simulink model "Simulink_5"  (R2016b)
settings: Solver=VariableStepAuto  StartTime=0.0  StopTime=50  RelTol=1e-3
values from neighbouring files (symbols this model uses):
  C_lat = [1 0 0 0 ... (first row only)    [ejercicio07_lateral_C.m]
  D_lat = zeros(2)    [ejercicio07_lateral_C.m]
  dt = 0.001    [ejercicio07_lateral_C.m]    (also in ejercicio07_longitudinal_C.m)
  F_lat = A_lat*Tm + I    [ejercicio07_lateral_C.m]
  G_lat = B_lat*Tm    [ejercicio07_lateral_C.m]
  Kc = Kc_a(:,1:4)    [ejercicio07_lateral_C.m]    (also in ejercicio07_longitudinal_C.m)
  Ki = -Kc_a(:,5:6)    [ejercicio07_lateral_C.m]    (also in ejercicio07_longitudinal_C.m)
  Ko_d = dlqe(F_lat,G_lat,C_lat,V1,V2)    [ejercicio07_lateral_C.m]    (also in ejercicio07_longitudinal_C.m = dlqe(F_lon,G_lon,C_lon,V1,V2))
  PreC = [Cyr*(I-Fyr)^(-1)*G_lat+D_lat]^(-1)    [ejercicio07_lateral_C.m]    (also in ejercicio07_longitudinal_C.m = [Cyr*(I-Fyr)^(-1)*G_lon+D_lon]^(-1))
  tau_a = 0.5    [ejercicio07_lateral_C.m]
  tau_r = 1/20    (= 0.05)    [ejercicio07_lateral_C.m]
  Tm = 0.003    [ejercicio07_lateral_C.m]    (also in ejercicio07_longitudinal_C.m)
undefined symbols (not defined in the file or in its folder): DiscIntNeverNeededParam, Ko
undefined symbols (not defined in the file): sys_lat
(part 1 of 2)
settings Model: Creator=mluser  LastModifiedBy=Alvaro
settings DataIOCC: ReturnWorkspaceOutputs=on
settings DebuggingCC: SFMachineParentedDataDiag=error
settings SFSimCC: SimUseLocalCustomCode=on
settings RTWCC: RTWUseLocalCustomCode=on

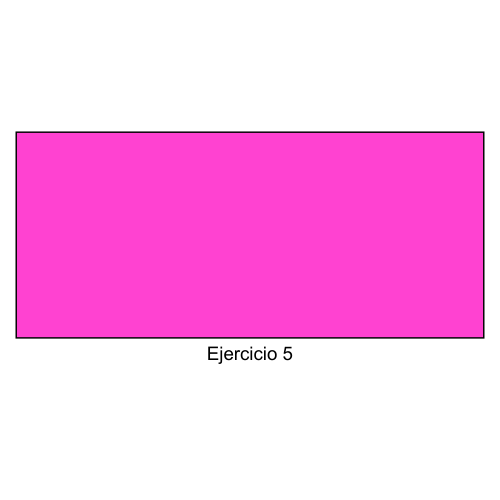
[thumbnail: Simulink's stored preview of the top-level diagram]
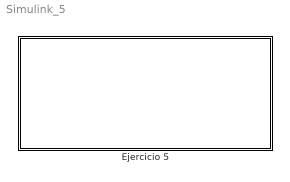
== system Simulink_5 ==
  Ejercicio 5 : Subsystem

== system Simulink_5/Ejercicio 5 ==
  EJERCICIO 5 CONTINUO : Subsystem  Commented=on
  EJERCICIO 5 DISCRETO : Subsystem  Commented=on

== system Simulink_5/Ejercicio 5/EJERCICIO 5 CONTINUO ==
  Control lateral con observador de estados %bien : Subsystem
  Control lateral con observador de estados sin perturbacion %bien : Subsystem
  Control laterall con accion integral %bien : Subsystem

== system Simulink_5/Ejercicio 5/EJERCICIO 5 DISCRETO ==
  COMPARATIVA : Subsystem
  CONTROL LATERAL DISCRETO : Subsystem  Commented=on
  CONTROL LATERAL DISCRETO ACCION INTEGRAL : Subsystem  Commented=on
  CONTROL LATERALDISCRETO FBW : Subsystem  Commented=on

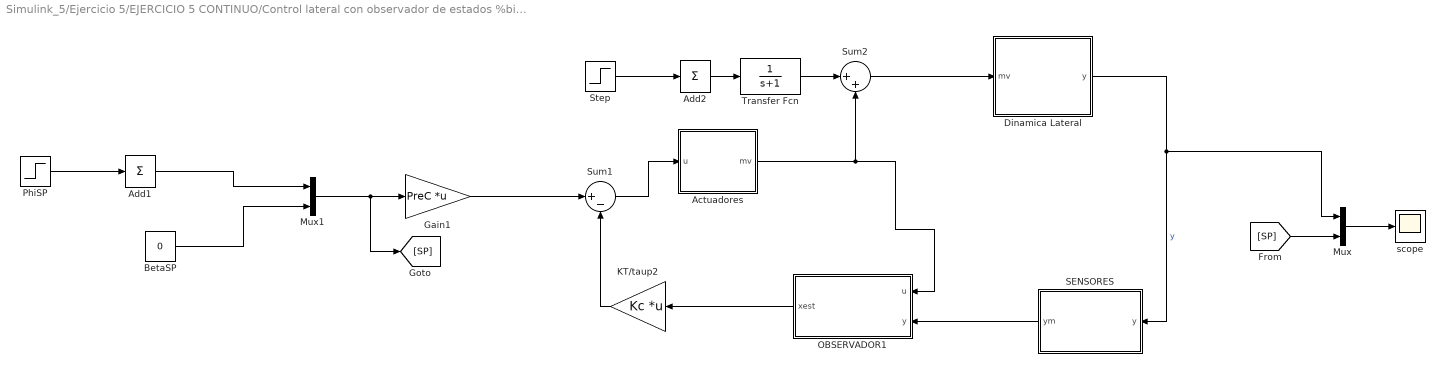
== system Simulink_5/Ejercicio 5/EJERCICIO 5 CONTINUO/Control lateral con observador de estados %bien ==
  Actuadores : Subsystem
  Add1 : Sum  Inputs=+
  Add2 : Sum  Inputs=+
  BetaSP : Constant  Value=0
  Dinamica Lateral : Subsystem  mask(Dinámica longitudinal F-16){A=sys_lat.a, B=sys_lat.b, C=sys_lat.c, D=sys_lat.d, X0=[0 0 0 0]}
      mask prompts: A "Matriz de estados (A)"; B "Matriz de entrada (B)"; C "Matriz de salida (C)"; D "Matriz de transmisión directa (D)"; X0 "Condiciones iniciales (nominales)"
      mask help: Modelo lineal de la dinámica longitudinal del F-16
  Gain1 : Gain  Gain=PreC  Multiplication=Matrix(K*u)
  KT/taup2 : Gain  Gain=Kc  Multiplication=Matrix(K*u)
  Mux : Mux  Inputs=2
  Mux1 : Mux  Inputs=2
  OBSERVADOR1 : Subsystem  mask(Dinámica longitudinal F-16){A=sys_lat.a, B=sys_lat.b, C=sys_lat.c, D=sys_lat.d, X0=[0 0 0 0], Ko=Ko}
      mask prompts: A "Matriz de estados (A)"; B "Matriz de entrada (B)"; C "Matriz de salida (C)"; D "Matriz de transmisión directa (D)"; X0 "Condiciones iniciales (nominales)"; Ko "Ganancia del observador"
      mask help: Modelo lineal de la dinámica longitudinal del F-16
  PhiSP : Step  Time=[5 25]  Before=[0 0]  After=[10 -10]  SampleTime=0
  SENSORES : Subsystem
  Step : Step  Time=[40 41]  After=[1 -1]  SampleTime=0
  Sum1 : Sum  Inputs=|+-
  Sum2 : Sum  Inputs=|++
  Transfer Fcn : TransferFcn  Denominator=[1 1]
  scope : Scope
  wires:
  Mux1/1 -> [SP], Gain1/1
  Gain1/1 -> Sum1/1
  Mux/1 -> scope/1
  [SP] -> Mux/2
  KT/taup2/1 -> Sum1/2
  SENSORES/1(ym) -> OBSERVADOR1/2(y)
  OBSERVADOR1/1(xest) -> KT/taup2/1
  Dinamica Lateral/1(y) -> Mux/1, SENSORES/1(y)  "y"
  PhiSP/1 -> Add1/1
  Add1/1 -> Mux1/1
  Actuadores/1(mv) -> OBSERVADOR1/1(u), Sum2/2
  Sum1/1 -> Actuadores/1(u)
  BetaSP/1 -> Mux1/2
  Step/1 -> Add2/1
  Transfer Fcn/1 -> Sum2/1
  Add2/1 -> Transfer Fcn/1
  Sum2/1 -> Dinamica Lateral/1(mv)

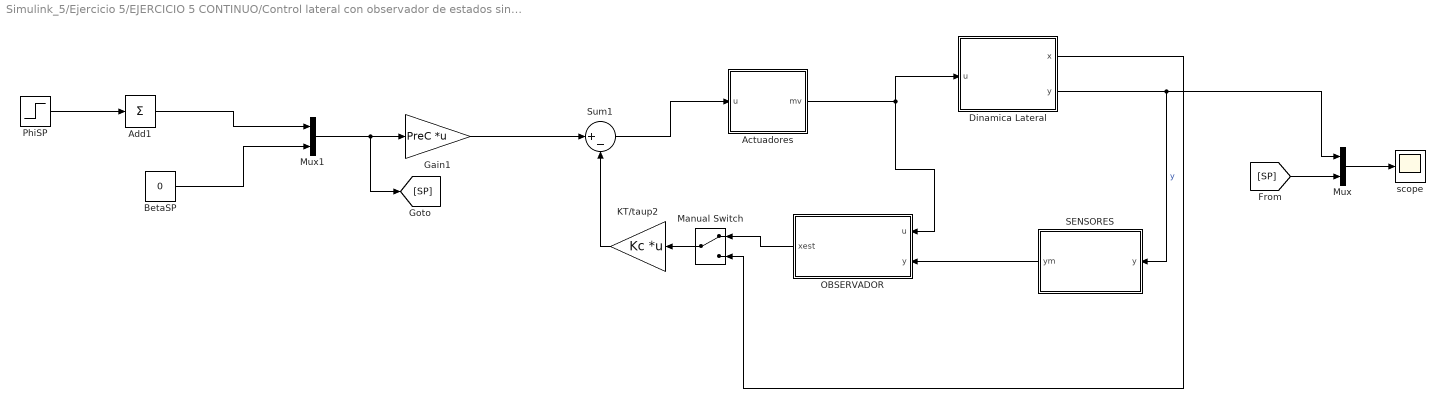
== system Simulink_5/Ejercicio 5/EJERCICIO 5 CONTINUO/Control lateral con observador de estados sin perturbacion %bien ==
  Actuadores : Subsystem
  Add1 : Sum  Inputs=+
  BetaSP : Constant  Value=0
  Dinamica Lateral : Subsystem  mask(Dinámica longitudinal F-16){A=sys_lat.a, B=sys_lat.b, C=sys_lat.c, D=sys_lat.d, X0=[0 0 0 0]}
      mask prompts: A "Matriz de estados (A)"; B "Matriz de entrada (B)"; C "Matriz de salida (C)"; D "Matriz de transmisión directa (D)"; X0 "Condiciones iniciales (nominales)"
      mask help: Modelo lineal de la dinámica longitudinal del F-16
  Gain1 : Gain  Gain=PreC  Multiplication=Matrix(K*u)
  KT/taup2 : Gain  Gain=Kc  Multiplication=Matrix(K*u)
  Manual Switch : ManualSwitch
  Mux : Mux  Inputs=2
  Mux1 : Mux  Inputs=2
  OBSERVADOR : Subsystem  mask(Dinámica longitudinal F-16){A=sys_lat.a, B=sys_lat.b, C=sys_lat.c, D=sys_lat.d, X0=[0 0 0 0], Ko=Ko}
      mask prompts: A "Matriz de estados (A)"; B "Matriz de entrada (B)"; C "Matriz de salida (C)"; D "Matriz de transmisión directa (D)"; X0 "Condiciones iniciales (nominales)"; Ko "Ganancia del observador"
      mask help: Modelo lineal de la dinámica longitudinal del F-16
  PhiSP : Step  Time=[5 25]  Before=[0 0]  After=[10 -10]  SampleTime=0
  SENSORES : Subsystem
  Sum1 : Sum  Inputs=|+-
  scope : Scope
  wires:
  Actuadores/1(mv) -> Dinamica Lateral/1(u), OBSERVADOR/1(u)
  [SP] -> Mux/2
  Dinamica Lateral/2(y) -> Mux/1, SENSORES/1(y)  "y"
  Add1/1 -> Mux1/1
  Mux/1 -> scope/1
  BetaSP/1 -> Mux1/2
  PhiSP/1 -> Add1/1
  Gain1/1 -> Sum1/1
  KT/taup2/1 -> Sum1/2
  Sum1/1 -> Actuadores/1(u)
  SENSORES/1(ym) -> OBSERVADOR/2(y)
  Mux1/1 -> [SP], Gain1/1
  Manual Switch/1 -> KT/taup2/1
  OBSERVADOR/1(xest) -> Manual Switch/1
  Dinamica Lateral/1(x) -> Manual Switch/2

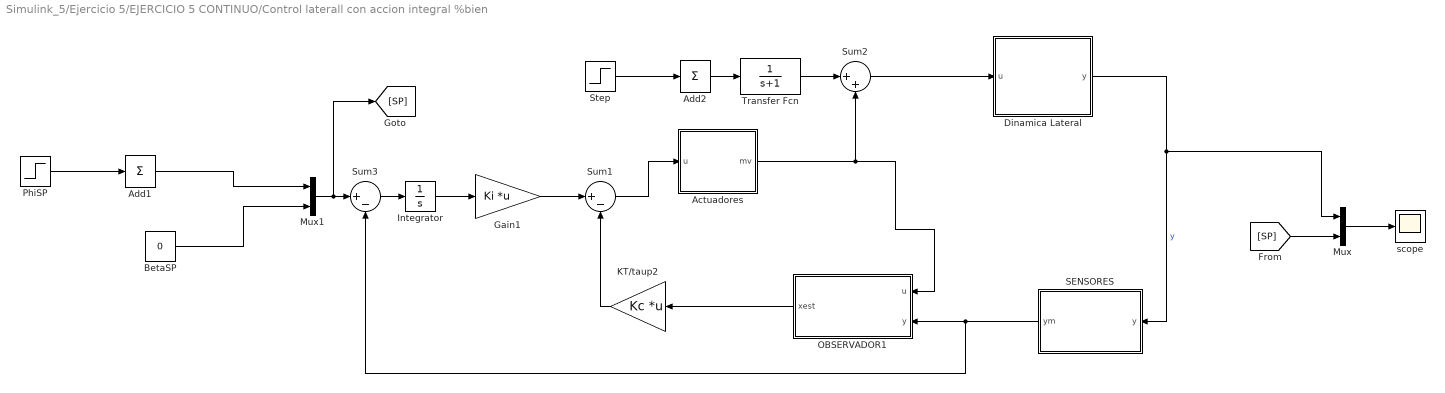
== system Simulink_5/Ejercicio 5/EJERCICIO 5 CONTINUO/Control laterall con accion integral %bien ==
  Actuadores : Subsystem
  Add1 : Sum  Inputs=+
  Add2 : Sum  Inputs=+
  BetaSP : Constant  Value=0
  Dinamica Lateral : Subsystem  mask(Dinámica longitudinal F-16){A=sys_lat.a, B=sys_lat.b, C=sys_lat.c, D=sys_lat.d, X0=[0 0 0 0]}
      mask prompts: A "Matriz de estados (A)"; B "Matriz de entrada (B)"; C "Matriz de salida (C)"; D "Matriz de transmisión directa (D)"; X0 "Condiciones iniciales (nominales)"
      mask help: Modelo lineal de la dinámica longitudinal del F-16
  Gain1 : Gain  Gain=Ki  Multiplication=Matrix(K*u)
  Integrator : Integrator
  KT/taup2 : Gain  Gain=Kc  Multiplication=Matrix(K*u)
  Mux : Mux  Inputs=2
  Mux1 : Mux  Inputs=2
  OBSERVADOR1 : Subsystem  mask(Dinámica longitudinal F-16){A=sys_lat.a, B=sys_lat.b, C=sys_lat.c, D=sys_lat.d, X0=[0 0 0 0], Ko=Ko}
      mask prompts: A "Matriz de estados (A)"; B "Matriz de entrada (B)"; C "Matriz de salida (C)"; D "Matriz de transmisión directa (D)"; X0 "Condiciones iniciales (nominales)"; Ko "Ganancia del observador"
      mask help: Modelo lineal de la dinámica longitudinal del F-16
  PhiSP : Step  Time=[5 25]  Before=[0 0]  After=[10 -10]  SampleTime=0
  SENSORES : Subsystem
  Step : Step  Time=[40 41]  After=[1 -1]  SampleTime=0
  Sum1 : Sum  Inputs=|+-
  Sum2 : Sum  Inputs=|++
  Sum3 : Sum  Inputs=|+-
  Transfer Fcn : TransferFcn  Denominator=[1 1]
  scope : Scope
  wires:
  Actuadores/1(mv) -> OBSERVADOR1/1(u), Sum2/2
  Dinamica Lateral/1(y) -> Mux/1, SENSORES/1(y)  "y"
  BetaSP/1 -> Mux1/2
  Add1/1 -> Mux1/1
  Sum2/1 -> Dinamica Lateral/1(u)
  KT/taup2/1 -> Sum1/2
  Gain1/1 -> Sum1/1
  Add2/1 -> Transfer Fcn/1
  Step/1 -> Add2/1
  PhiSP/1 -> Add1/1
  SENSORES/1(ym) -> OBSERVADOR1/2(y), Sum3/2
  Mux/1 -> scope/1
  Sum1/1 -> Actuadores/1(u)
  [SP] -> Mux/2
  OBSERVADOR1/1(xest) -> KT/taup2/1
  Transfer Fcn/1 -> Sum2/1
  Mux1/1 -> [SP], Sum3/1
  Integrator/1 -> Gain1/1
  Sum3/1 -> Integrator/1

== system Simulink_5/Ejercicio 5/EJERCICIO 5 DISCRETO/COMPARATIVA ==
  Comparativa Integral : Subsystem  Commented=on
  Comparativa modal : Subsystem

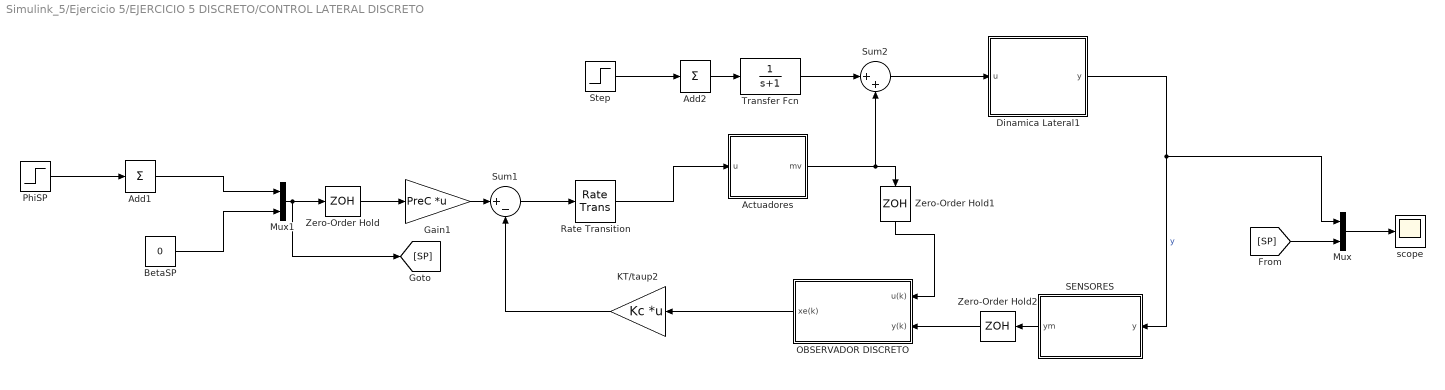
== system Simulink_5/Ejercicio 5/EJERCICIO 5 DISCRETO/CONTROL LATERAL DISCRETO ==
  Actuadores : Subsystem
  Add1 : Sum  Inputs=+
  Add2 : Sum  Inputs=+
  BetaSP : Constant  Value=0
  Dinamica Lateral1 : Subsystem  mask(Dinámica longitudinal F-16){A=sys_lat.a, B=sys_lat.b, C=sys_lat.c, D=sys_lat.d, X0=[0 0 0 0]}
      mask prompts: A "Matriz de estados (A)"; B "Matriz de entrada (B)"; C "Matriz de salida (C)"; D "Matriz de transmisión directa (D)"; X0 "Condiciones iniciales (nominales)"
      mask help: Modelo lineal de la dinámica longitudinal del F-16
  Gain1 : Gain  Gain=PreC  Multiplication=Matrix(K*u)
  KT/taup2 : Gain  Gain=Kc  Multiplication=Matrix(K*u)
  Mux : Mux  Inputs=2
  Mux1 : Mux  Inputs=2
  OBSERVADOR DISCRETO : Subsystem  mask(Dinámica longitudinal F-16){F=F_lat, G=G_lat, C=C_lat, D=D_lat, Ko=Ko_d}
      mask prompts: F "Matriz de estados (A)"; G "Matriz de entrada (B)"; C "Matriz de salida (C)"; D "Matriz de transmisión directa (D)"; Ko "Ganancia del observador"
      mask help: Modelo lineal de la dinámica longitudinal del F-16
  PhiSP : Step  Time=[5 25]  Before=[0 0]  After=[10 -10]  SampleTime=0
  Rate Transition : RateTransition
  SENSORES : Subsystem
  Step : Step  Time=[40 41]  After=[1 -1]  SampleTime=0
  Sum1 : Sum  Inputs=|+-
  Sum2 : Sum  Inputs=|++
  Transfer Fcn : TransferFcn  Denominator=[1 1]
  Zero-Order Hold : ZeroOrderHold  SampleTime=-1
  Zero-Order Hold1 : ZeroOrderHold  SampleTime=-1
  Zero-Order Hold2 : ZeroOrderHold  SampleTime=-1
  scope : Scope
  wires:
  Actuadores/1(mv) -> Zero-Order Hold1/1, Sum2/2
  Mux1/1 -> Zero-Order Hold/1, [SP]
  [SP] -> Mux/2
  Add1/1 -> Mux1/1
  OBSERVADOR DISCRETO/1(xe(k)) -> KT/taup2/1
  SENSORES/1(ym) -> Zero-Order Hold2/1
  KT/taup2/1 -> Sum1/2
  PhiSP/1 -> Add1/1
  Gain1/1 -> Sum1/1
  Mux/1 -> scope/1
  BetaSP/1 -> Mux1/2
  Dinamica Lateral1/1(y) -> SENSORES/1(y), Mux/1  "y"
  Zero-Order Hold/1 -> Gain1/1
  Rate Transition/1 -> Actuadores/1(u)
  Sum1/1 -> Rate Transition/1
  Zero-Order Hold1/1 -> OBSERVADOR DISCRETO/1(u(k))
  Zero-Order Hold2/1 -> OBSERVADOR DISCRETO/2(y(k))
  Add2/1 -> Transfer Fcn/1
  Step/1 -> Add2/1
  Transfer Fcn/1 -> Sum2/1
  Sum2/1 -> Dinamica Lateral1/1(u)

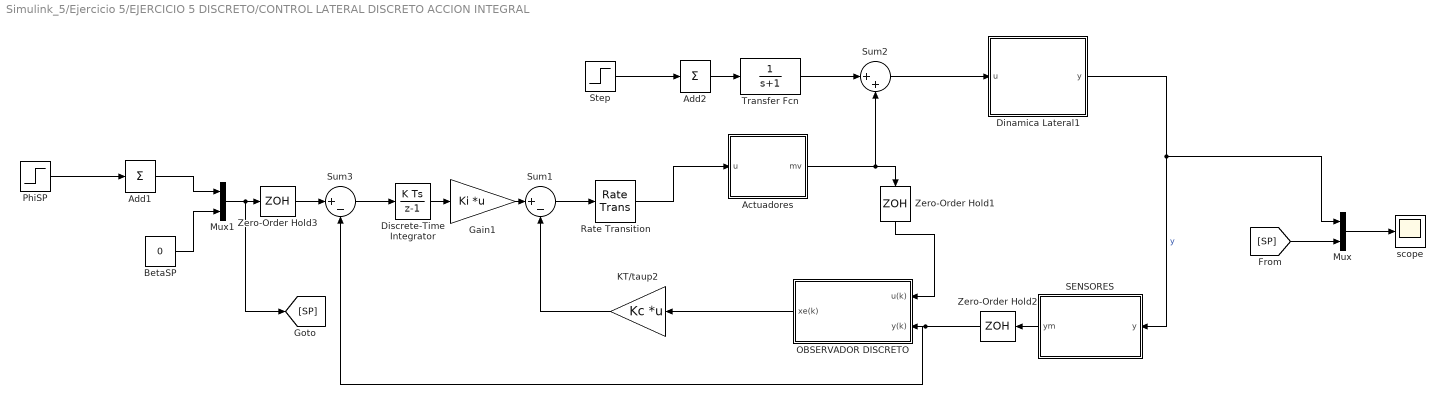
== system Simulink_5/Ejercicio 5/EJERCICIO 5 DISCRETO/CONTROL LATERAL DISCRETO ACCION INTEGRAL ==
  Actuadores : Subsystem
  Add1 : Sum  Inputs=+
  Add2 : Sum  Inputs=+
  BetaSP : Constant  Value=0
  Dinamica Lateral1 : Subsystem  mask(Dinámica longitudinal F-16){A=sys_lat.a, B=sys_lat.b, C=sys_lat.c, D=sys_lat.d, X0=[0 0 0 0]}
      mask prompts: A "Matriz de estados (A)"; B "Matriz de entrada (B)"; C "Matriz de salida (C)"; D "Matriz de transmisión directa (D)"; X0 "Condiciones iniciales (nominales)"
      mask help: Modelo lineal de la dinámica longitudinal del F-16
  Discrete-Time Integrator : DiscreteIntegrator  InitialConditionSetting=State (most efficient)  SampleTime=-1  ICPrevOutput=DiscIntNeverNeededParam  ICPrevScaledInput=DiscIntNeverNeededParam
  Gain1 : Gain  Gain=Ki  Multiplication=Matrix(K*u)
  KT/taup2 : Gain  Gain=Kc  Multiplication=Matrix(K*u)
  Mux : Mux  Inputs=2
  Mux1 : Mux  Inputs=2
  OBSERVADOR DISCRETO : Subsystem  mask(Dinámica longitudinal F-16){F=F_lat, G=G_lat, C=C_lat, D=D_lat, Ko=Ko_d}
      mask prompts: F "Matriz de estados (A)"; G "Matriz de entrada (B)"; C "Matriz de salida (C)"; D "Matriz de transmisión directa (D)"; Ko "Ganancia del observador"
      mask help: Modelo lineal de la dinámica longitudinal del F-16
  PhiSP : Step  Time=[5 25]  Before=[0 0]  After=[10 -10]  SampleTime=0
  Rate Transition : RateTransition
  SENSORES : Subsystem
  Step : Step  Time=[40 41]  After=[1 -1]  SampleTime=0
  Sum1 : Sum  Inputs=|+-
  Sum2 : Sum  Inputs=|++
  Sum3 : Sum  Inputs=|+-
  Transfer Fcn : TransferFcn  Denominator=[1 1]
  Zero-Order Hold1 : ZeroOrderHold  SampleTime=-1
  Zero-Order Hold2 : ZeroOrderHold  SampleTime=-1
  Zero-Order Hold3 : ZeroOrderHold  SampleTime=-1
  scope : Scope
  wires:
  Zero-Order Hold2/1 -> Sum3/2, OBSERVADOR DISCRETO/2(y(k))
  Rate Transition/1 -> Actuadores/1(u)
  Mux1/1 -> Zero-Order Hold3/1, [SP]
  Dinamica Lateral1/1(y) -> SENSORES/1(y), Mux/1  "y"
  [SP] -> Mux/2
  Add2/1 -> Transfer Fcn/1
  Gain1/1 -> Sum1/1
  Discrete-Time Integrator/1 -> Gain1/1
  SENSORES/1(ym) -> Zero-Order Hold2/1
  Transfer Fcn/1 -> Sum2/1
  Step/1 -> Add2/1
  KT/taup2/1 -> Sum1/2
  BetaSP/1 -> Mux1/2
  Sum1/1 -> Rate Transition/1
  OBSERVADOR DISCRETO/1(xe(k)) -> KT/taup2/1
  Add1/1 -> Mux1/1
  Actuadores/1(mv) -> Zero-Order Hold1/1, Sum2/2
  PhiSP/1 -> Add1/1
  Mux/1 -> scope/1
  Sum2/1 -> Dinamica Lateral1/1(u)
  Zero-Order Hold1/1 -> OBSERVADOR DISCRETO/1(u(k))
  Sum3/1 -> Discrete-Time Integrator/1
  Zero-Order Hold3/1 -> Sum3/1

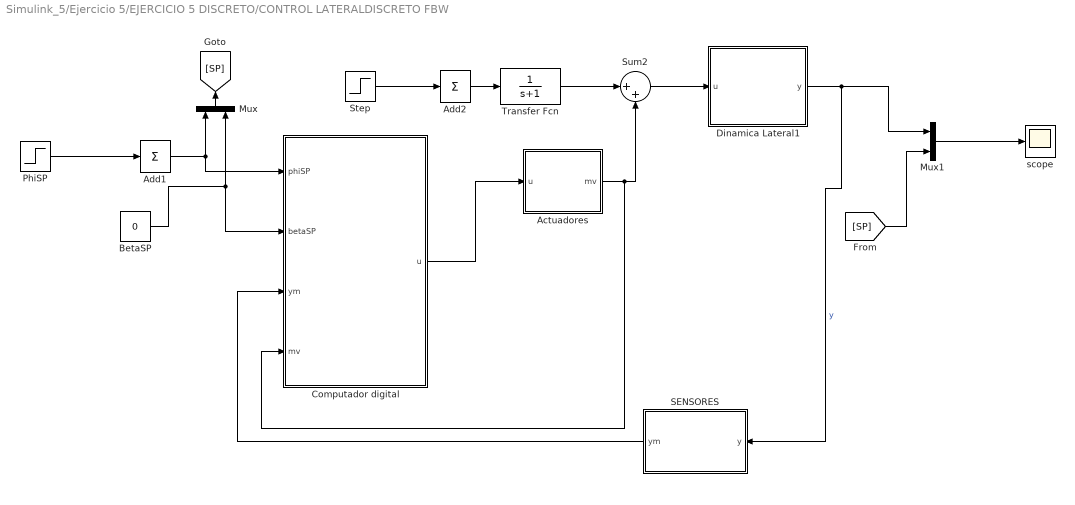
== system Simulink_5/Ejercicio 5/EJERCICIO 5 DISCRETO/CONTROL LATERALDISCRETO FBW ==
  Actuadores : Subsystem
  Add1 : Sum  Inputs=+
  Add2 : Sum  Inputs=+
  BetaSP : Constant  Value=0
  Computador digital : Subsystem
  Dinamica Lateral1 : Subsystem  mask(Dinámica longitudinal F-16){A=sys_lat.a, B=sys_lat.b, C=sys_lat.c, D=sys_lat.d, X0=[0 0 0 0]}
      mask prompts: A "Matriz de estados (A)"; B "Matriz de entrada (B)"; C "Matriz de salida (C)"; D "Matriz de transmisión directa (D)"; X0 "Condiciones iniciales (nominales)"
      mask help: Modelo lineal de la dinámica longitudinal del F-16
  Mux : Mux  Inputs=2
  Mux1 : Mux  Inputs=2
  PhiSP : Step  Time=[5 25]  Before=[0 0]  After=[10 -10]  SampleTime=0
  SENSORES : Subsystem
  Step : Step  Time=[40 41]  After=[1 -1]  SampleTime=0
  Sum2 : Sum  Inputs=|++
  Transfer Fcn : TransferFcn  Denominator=[1 1]
  scope : Scope
  wires:
  Add1/1 -> Computador digital/1(phiSP), Mux/1
  BetaSP/1 -> Computador digital/2(betaSP), Mux/2
  PhiSP/1 -> Add1/1
  Transfer Fcn/1 -> Sum2/1
  Add2/1 -> Transfer Fcn/1
  Sum2/1 -> Dinamica Lateral1/1(u)
  Step/1 -> Add2/1
  Actuadores/1(mv) -> Computador digital/4(mv), Sum2/2
  Mux/1 -> [SP]
  Mux1/1 -> scope/1
  [SP] -> Mux1/2
  Dinamica Lateral1/1(y) -> SENSORES/1(y), Mux1/1  "y"
  Computador digital/1(u) -> Actuadores/1(u)
  SENSORES/1(ym) -> Computador digital/3(ym)

== system Simulink_5/Ejercicio 5/EJERCICIO 5 CONTINUO/Control lateral con observador de estados %bien/Actuadores ==
  u : Inport
  Aleron : Subsystem
  Demux : Demux  Outputs=2
  Mux2 : Mux  Inputs=2
  Scope : Scope
  TIMÓN : Subsystem
  mv : Outport
  wires:
  u/1 -> Demux/1
  Mux2/1 -> mv/1, Scope/1
  Demux/1 -> Aleron/1(u_a)
  Demux/2 -> TIMÓN/1(u_r)
  Aleron/1(delta_a) -> Mux2/1
  TIMÓN/1(delta_r) -> Mux2/2

== system Simulink_5/Ejercicio 5/EJERCICIO 5 CONTINUO/Control lateral con observador de estados %bien/Dinamica Lateral ==
  mv : Inport
  Integrator5 : Integrator
  Km1 : Gain  Gain=D  Multiplication=Matrix(K*u)
  Km10 : Gain  Gain=A  Multiplication=Matrix(K*u)
  Km2 : Gain  Gain=C  Multiplication=Matrix(K*u)
  Km8 : Gain  Gain=B  Multiplication=Matrix(K*u)
  Sum1 : Sum  Inputs=++|
  Sum12 : Sum  Inputs=|++
  y : Outport
  wires:
  Km8/1 -> Sum12/1
  Sum12/1 -> Integrator5/1
  Integrator5/1 -> Km10/1, Km2/1  "x"
  Km10/1 -> Sum12/2
  Km2/1 -> Sum1/2
  Km1/1 -> Sum1/1
  Sum1/1 -> y/1
  mv/1 -> Km8/1, Km1/1

== system Simulink_5/Ejercicio 5/EJERCICIO 5 CONTINUO/Control lateral con observador de estados %bien/OBSERVADOR1 ==
  u : Inport
  y : Inport  Port=2
  Integrator5 : Integrator
  Km1 : Gain  Gain=D  Multiplication=Matrix(K*u)
  Km10 : Gain  Gain=A  Multiplication=Matrix(K*u)
  Km2 : Gain  Gain=C  Multiplication=Matrix(K*u)
  Km3 : Gain  Gain=Ko  Multiplication=Matrix(K*u)
  Km8 : Gain  Gain=B  Multiplication=Matrix(K*u)
  Sum1 : Sum  Inputs=++|
  Sum12 : Sum  Inputs=+++
  Sum2 : Sum  Inputs=+-|
  xest : Outport
  wires:
  Km8/1 -> Sum12/1
  Sum12/1 -> Integrator5/1
  Integrator5/1 -> Km2/1, Km10/1, xest/1  "xe"
  Km10/1 -> Sum12/3
  Km2/1 -> Sum1/2
  Km1/1 -> Sum1/1
  Sum1/1 -> Sum2/2  "ye"
  u/1 -> Km8/1, Km1/1
  y/1 -> Sum2/1
  Sum2/1 -> Km3/1
  Km3/1 -> Sum12/2

== system Simulink_5/Ejercicio 5/EJERCICIO 5 CONTINUO/Control lateral con observador de estados %bien/SENSORES ==
  y : Inport
  Add2 : Sum
  Add3 : Sum
  Demux : Demux  Outputs=2
  Mux2 : Mux  Inputs=2
  Ruido de medida1 : RandomNumber  Variance=1e-6  Seed=123456  SampleTime=dt
  Ruido de medida2 : RandomNumber  Variance=1e-6  Seed=123456  SampleTime=dt
  ym : Outport
  wires:
  y/1 -> Demux/1
  Ruido de medida1/1 -> Add2/1
  Add2/1 -> Mux2/1
  Demux/1 -> Add2/2
  Mux2/1 -> ym/1
  Demux/2 -> Add3/1
  Add3/1 -> Mux2/2
  Ruido de medida2/1 -> Add3/2

== system Simulink_5/Ejercicio 5/EJERCICIO 5 CONTINUO/Control lateral con observador de estados sin perturbacion %bien/Actuadores ==
  u : Inport
  Aleron : Subsystem
  Demux : Demux  Outputs=2
  Mux2 : Mux  Inputs=2
  Scope : Scope
  TIMÓN : Subsystem
  mv : Outport
  wires:
  u/1 -> Demux/1
  Mux2/1 -> mv/1, Scope/1
  Demux/1 -> Aleron/1(u_a)
  Demux/2 -> TIMÓN/1(u_r)
  Aleron/1(delta_a) -> Mux2/1
  TIMÓN/1(delta_r) -> Mux2/2

== system Simulink_5/Ejercicio 5/EJERCICIO 5 CONTINUO/Control lateral con observador de estados sin perturbacion %bien/Dinamica Lateral ==
  u : Inport
  Integrator5 : Integrator
  Km1 : Gain  Gain=D  Multiplication=Matrix(K*u)
  Km10 : Gain  Gain=A  Multiplication=Matrix(K*u)
  Km2 : Gain  Gain=C  Multiplication=Matrix(K*u)
  Km8 : Gain  Gain=B  Multiplication=Matrix(K*u)
  Sum1 : Sum  Inputs=++|
  Sum12 : Sum  Inputs=|++
  x : Outport
  y : Outport  Port=2
  wires:
  Km8/1 -> Sum12/1
  Sum12/1 -> Integrator5/1
  Integrator5/1 -> x/1, Km10/1, Km2/1  "x"
  Km10/1 -> Sum12/2
  Km2/1 -> Sum1/2
  Km1/1 -> Sum1/1
  Sum1/1 -> y/1
  u/1 -> Km8/1, Km1/1

== system Simulink_5/Ejercicio 5/EJERCICIO 5 CONTINUO/Control lateral con observador de estados sin perturbacion %bien/OBSERVADOR ==
  u : Inport
  y : Inport  Port=2
  Integrator5 : Integrator
  Km1 : Gain  Gain=D  Multiplication=Matrix(K*u)
  Km10 : Gain  Gain=A  Multiplication=Matrix(K*u)
  Km2 : Gain  Gain=C  Multiplication=Matrix(K*u)
  Km3 : Gain  Gain=Ko  Multiplication=Matrix(K*u)
  Km8 : Gain  Gain=B  Multiplication=Matrix(K*u)
  Sum1 : Sum  Inputs=++|
  Sum12 : Sum  Inputs=+++
  Sum2 : Sum  Inputs=+-|
  xest : Outport
  wires:
  Km8/1 -> Sum12/1
  Sum12/1 -> Integrator5/1
  Integrator5/1 -> Km2/1, Km10/1, xest/1  "xe"
  Km10/1 -> Sum12/3
  Km2/1 -> Sum1/2
  Km1/1 -> Sum1/1
  Sum1/1 -> Sum2/2  "ye"
  u/1 -> Km8/1, Km1/1
  y/1 -> Sum2/1
  Sum2/1 -> Km3/1
  Km3/1 -> Sum12/2

== system Simulink_5/Ejercicio 5/EJERCICIO 5 CONTINUO/Control lateral con observador de estados sin perturbacion %bien/SENSORES ==
  y : Inport
  Add2 : Sum
  Add3 : Sum
  Demux : Demux  Outputs=2
  Mux2 : Mux  Inputs=2
  Ruido de medida1 : RandomNumber  Variance=1e-6  Seed=123456  SampleTime=dt
  Ruido de medida2 : RandomNumber  Variance=1e-6  Seed=123456  SampleTime=dt
  ym : Outport
  wires:
  y/1 -> Demux/1
  Ruido de medida1/1 -> Add2/1
  Add2/1 -> Mux2/1
  Demux/1 -> Add2/2
  Mux2/1 -> ym/1
  Demux/2 -> Add3/1
  Add3/1 -> Mux2/2
  Ruido de medida2/1 -> Add3/2

== system Simulink_5/Ejercicio 5/EJERCICIO 5 CONTINUO/Control laterall con accion integral %bien/Actuadores ==
  u : Inport
  Aleron : Subsystem
  Demux : Demux  Outputs=2
  Mux2 : Mux  Inputs=2
  Scope : Scope
  TIMÓN : Subsystem
  mv : Outport
  wires:
  u/1 -> Demux/1
  Mux2/1 -> mv/1, Scope/1
  Demux/1 -> Aleron/1(u_a)
  Demux/2 -> TIMÓN/1(u_r)
  Aleron/1(delta_a) -> Mux2/1
  TIMÓN/1(delta_r) -> Mux2/2

== system Simulink_5/Ejercicio 5/EJERCICIO 5 CONTINUO/Control laterall con accion integral %bien/Dinamica Lateral ==
  u : Inport
  Integrator5 : Integrator
  Km1 : Gain  Gain=D  Multiplication=Matrix(K*u)
  Km10 : Gain  Gain=A  Multiplication=Matrix(K*u)
  Km2 : Gain  Gain=C  Multiplication=Matrix(K*u)
  Km8 : Gain  Gain=B  Multiplication=Matrix(K*u)
  Sum1 : Sum  Inputs=++|
  Sum12 : Sum  Inputs=|++
  y : Outport
  wires:
  Km8/1 -> Sum12/1
  Sum12/1 -> Integrator5/1
  Integrator5/1 -> Km10/1, Km2/1  "x"
  Km10/1 -> Sum12/2
  Km2/1 -> Sum1/2
  Km1/1 -> Sum1/1
  Sum1/1 -> y/1
  u/1 -> Km8/1, Km1/1

== system Simulink_5/Ejercicio 5/EJERCICIO 5 CONTINUO/Control laterall con accion integral %bien/OBSERVADOR1 ==
  u : Inport
  y : Inport  Port=2
  Integrator5 : Integrator
  Km1 : Gain  Gain=D  Multiplication=Matrix(K*u)
  Km10 : Gain  Gain=A  Multiplication=Matrix(K*u)
  Km2 : Gain  Gain=C  Multiplication=Matrix(K*u)
  Km3 : Gain  Gain=Ko  Multiplication=Matrix(K*u)
  Km8 : Gain  Gain=B  Multiplication=Matrix(K*u)
  Sum1 : Sum  Inputs=++|
  Sum12 : Sum  Inputs=+++
  Sum2 : Sum  Inputs=+-|
  xest : Outport
  wires:
  Km8/1 -> Sum12/1
  Sum12/1 -> Integrator5/1
  Integrator5/1 -> Km2/1, Km10/1, xest/1  "xe"
  Km10/1 -> Sum12/3
  Km2/1 -> Sum1/2
  Km1/1 -> Sum1/1
  Sum1/1 -> Sum2/2  "ye"
  u/1 -> Km8/1, Km1/1
  y/1 -> Sum2/1
  Sum2/1 -> Km3/1
  Km3/1 -> Sum12/2

== system Simulink_5/Ejercicio 5/EJERCICIO 5 CONTINUO/Control laterall con accion integral %bien/SENSORES ==
  y : Inport
  Add2 : Sum
  Add3 : Sum
  Demux : Demux  Outputs=2
  Mux2 : Mux  Inputs=2
  Ruido de medida1 : RandomNumber  Variance=1e-6  Seed=123456  SampleTime=dt
  Ruido de medida2 : RandomNumber  Variance=1e-6  Seed=123456  SampleTime=dt
  ym : Outport
  wires:
  y/1 -> Demux/1
  Ruido de medida1/1 -> Add2/1
  Add2/1 -> Mux2/1
  Demux/1 -> Add2/2
  Mux2/1 -> ym/1
  Demux/2 -> Add3/1
  Add3/1 -> Mux2/2
  Ruido de medida2/1 -> Add3/2

== system Simulink_5/Ejercicio 5/EJERCICIO 5 DISCRETO/COMPARATIVA/Comparativa Integral ==
  CONTROL LATERAL DISCRETO ACCION INTEGRAL %bien : Subsystem
  Control laterall con accion integral %bien : Subsystem
  Mux : Mux  Inputs=2
  Scope : Scope
  wires:
  Control laterall con accion integral %bien/1(CONTINUA) -> Mux/1
  CONTROL LATERAL DISCRETO ACCION INTEGRAL %bien/1(Out1) -> Mux/2
  Mux/1 -> Scope/1

== system Simulink_5/Ejercicio 5/EJERCICIO 5 DISCRETO/COMPARATIVA/Comparativa modal ==
  CONTROL LATERAL DISCRETO %bien : Subsystem
  Control lateral con observador de estados %bien : Subsystem
  Mux : Mux  Inputs=2
  scope : Scope
  wires:
  Mux/1 -> scope/1
  CONTROL LATERAL DISCRETO %bien/1(DISCRETA) -> Mux/2
  Control lateral con observador de estados %bien/1(CONTINUA) -> Mux/1

== system Simulink_5/Ejercicio 5/EJERCICIO 5 DISCRETO/CONTROL LATERAL DISCRETO/Actuadores ==
  u : Inport
  Aleron : Subsystem
  Demux : Demux  Outputs=2
  Mux2 : Mux  Inputs=2
  Scope : Scope
  TIMÓN : Subsystem
  mv : Outport
  wires:
  u/1 -> Demux/1
  Mux2/1 -> mv/1, Scope/1
  Demux/1 -> Aleron/1(u_a)
  Demux/2 -> TIMÓN/1(u_r)
  Aleron/1(delta_a) -> Mux2/1
  TIMÓN/1(delta_r) -> Mux2/2

== system Simulink_5/Ejercicio 5/EJERCICIO 5 DISCRETO/CONTROL LATERAL DISCRETO/Dinamica Lateral1 ==
  u : Inport
  Integrator5 : Integrator
  Km1 : Gain  Gain=D  Multiplication=Matrix(K*u)
  Km10 : Gain  Gain=A  Multiplication=Matrix(K*u)
  Km2 : Gain  Gain=C  Multiplication=Matrix(K*u)
  Km8 : Gain  Gain=B  Multiplication=Matrix(K*u)
  Sum1 : Sum  Inputs=++|
  Sum12 : Sum  Inputs=|++
  y : Outport
  wires:
  Km8/1 -> Sum12/1
  Sum12/1 -> Integrator5/1
  Integrator5/1 -> Km10/1, Km2/1  "x"
  Km10/1 -> Sum12/2
  Km2/1 -> Sum1/2
  Km1/1 -> Sum1/1
  Sum1/1 -> y/1
  u/1 -> Km8/1, Km1/1

== system Simulink_5/Ejercicio 5/EJERCICIO 5 DISCRETO/CONTROL LATERAL DISCRETO/OBSERVADOR DISCRETO ==
  u(k) : Inport
  y(k) : Inport  Port=2
  Km1 : Gain  Gain=D  Multiplication=Matrix(K*u)
  Km10 : Gain  Gain=F  Multiplication=Matrix(K*u)
  Km2 : Gain  Gain=C  Multiplication=Matrix(K*u)
  Km3 : Gain  Gain=Ko  Multiplication=Matrix(K*u)
  Km8 : Gain  Gain=G  Multiplication=Matrix(K*u)
  Sum1 : Sum  Inputs=++|
  Sum12 : Sum  Inputs=+++
  Sum2 : Sum  Inputs=+-|
  Unit Delay : UnitDelay  SampleTime=Tm  HasFrameUpgradeWarning=on
  xe(k) : Outport
  wires:
  Km8/1 -> Sum12/1
  Sum12/1 -> Unit Delay/1  "xe(k+1)"
  Unit Delay/1 -> Km2/1, Km10/1, xe(k)/1  "xe(k)"
  Km10/1 -> Sum12/3
  Km2/1 -> Sum1/2
  Km1/1 -> Sum1/1
  Sum1/1 -> Sum2/2  "ye(k)"
  u(k)/1 -> Km8/1, Km1/1
  y(k)/1 -> Sum2/1
  Sum2/1 -> Km3/1
  Km3/1 -> Sum12/2

== system Simulink_5/Ejercicio 5/EJERCICIO 5 DISCRETO/CONTROL LATERAL DISCRETO/SENSORES ==
  y : Inport
  Add2 : Sum
  Add3 : Sum
  Demux : Demux  Outputs=2
  Mux2 : Mux  Inputs=2
  Ruido de medida1 : RandomNumber  Variance=1e-6  Seed=123456  SampleTime=dt
  Ruido de medida2 : RandomNumber  Variance=1e-6  Seed=123456  SampleTime=dt
  ym : Outport
  wires:
  y/1 -> Demux/1
  Ruido de medida1/1 -> Add2/1
  Add2/1 -> Mux2/1
  Demux/1 -> Add2/2
  Mux2/1 -> ym/1
  Demux/2 -> Add3/1
  Add3/1 -> Mux2/2
  Ruido de medida2/1 -> Add3/2

== system Simulink_5/Ejercicio 5/EJERCICIO 5 DISCRETO/CONTROL LATERAL DISCRETO ACCION INTEGRAL/Actuadores ==
  u : Inport
  Aleron : Subsystem
  Demux : Demux  Outputs=2
  Mux2 : Mux  Inputs=2
  Scope : Scope
  TIMÓN : Subsystem
  mv : Outport
  wires:
  u/1 -> Demux/1
  Mux2/1 -> mv/1, Scope/1
  Demux/1 -> Aleron/1(u_a)
  Demux/2 -> TIMÓN/1(u_r)
  Aleron/1(delta_a) -> Mux2/1
  TIMÓN/1(delta_r) -> Mux2/2

== system Simulink_5/Ejercicio 5/EJERCICIO 5 DISCRETO/CONTROL LATERAL DISCRETO ACCION INTEGRAL/Dinamica Lateral1 ==
  u : Inport
  Integrator5 : Integrator
  Km1 : Gain  Gain=D  Multiplication=Matrix(K*u)
  Km10 : Gain  Gain=A  Multiplication=Matrix(K*u)
  Km2 : Gain  Gain=C  Multiplication=Matrix(K*u)
  Km8 : Gain  Gain=B  Multiplication=Matrix(K*u)
  Sum1 : Sum  Inputs=++|
  Sum12 : Sum  Inputs=|++
  y : Outport
  wires:
  Km8/1 -> Sum12/1
  Sum12/1 -> Integrator5/1
  Integrator5/1 -> Km10/1, Km2/1  "x"
  Km10/1 -> Sum12/2
  Km2/1 -> Sum1/2
  Km1/1 -> Sum1/1
  Sum1/1 -> y/1
  u/1 -> Km8/1, Km1/1

== system Simulink_5/Ejercicio 5/EJERCICIO 5 DISCRETO/CONTROL LATERAL DISCRETO ACCION INTEGRAL/OBSERVADOR DISCRETO ==
  u(k) : Inport
  y(k) : Inport  Port=2
  Km1 : Gain  Gain=D  Multiplication=Matrix(K*u)
  Km10 : Gain  Gain=F  Multiplication=Matrix(K*u)
  Km2 : Gain  Gain=C  Multiplication=Matrix(K*u)
  Km3 : Gain  Gain=Ko  Multiplication=Matrix(K*u)
  Km8 : Gain  Gain=G  Multiplication=Matrix(K*u)
  Sum1 : Sum  Inputs=++|
  Sum12 : Sum  Inputs=+++
  Sum2 : Sum  Inputs=+-|
  Unit Delay : UnitDelay  SampleTime=Tm  HasFrameUpgradeWarning=on
  xe(k) : Outport
  wires:
  Km8/1 -> Sum12/1
  Sum12/1 -> Unit Delay/1  "xe(k+1)"
  Unit Delay/1 -> Km2/1, Km10/1, xe(k)/1  "xe(k)"
  Km10/1 -> Sum12/3
  Km2/1 -> Sum1/2
  Km1/1 -> Sum1/1
  Sum1/1 -> Sum2/2  "ye(k)"
  u(k)/1 -> Km8/1, Km1/1
  y(k)/1 -> Sum2/1
  Sum2/1 -> Km3/1
  Km3/1 -> Sum12/2

== system Simulink_5/Ejercicio 5/EJERCICIO 5 DISCRETO/CONTROL LATERAL DISCRETO ACCION INTEGRAL/SENSORES ==
  y : Inport
  Add2 : Sum
  Add3 : Sum
  Demux : Demux  Outputs=2
  Mux2 : Mux  Inputs=2
  Ruido de medida1 : RandomNumber  Variance=1e-6  Seed=123456  SampleTime=dt
  Ruido de medida2 : RandomNumber  Variance=1e-6  Seed=123456  SampleTime=dt
  ym : Outport
  wires:
  y/1 -> Demux/1
  Ruido de medida1/1 -> Add2/1
  Add2/1 -> Mux2/1
  Demux/1 -> Add2/2
  Mux2/1 -> ym/1
  Demux/2 -> Add3/1
  Add3/1 -> Mux2/2
  Ruido de medida2/1 -> Add3/2

== system Simulink_5/Ejercicio 5/EJERCICIO 5 DISCRETO/CONTROL LATERALDISCRETO FBW/Actuadores ==
  u : Inport
  Aleron : Subsystem
  Demux : Demux  Outputs=2
  Mux2 : Mux  Inputs=2
  Scope : Scope
  TIMÓN : Subsystem
  mv : Outport
  wires:
  u/1 -> Demux/1
  Mux2/1 -> mv/1, Scope/1
  Demux/1 -> Aleron/1(u_a)
  Demux/2 -> TIMÓN/1(u_r)
  Aleron/1(delta_a) -> Mux2/1
  TIMÓN/1(delta_r) -> Mux2/2

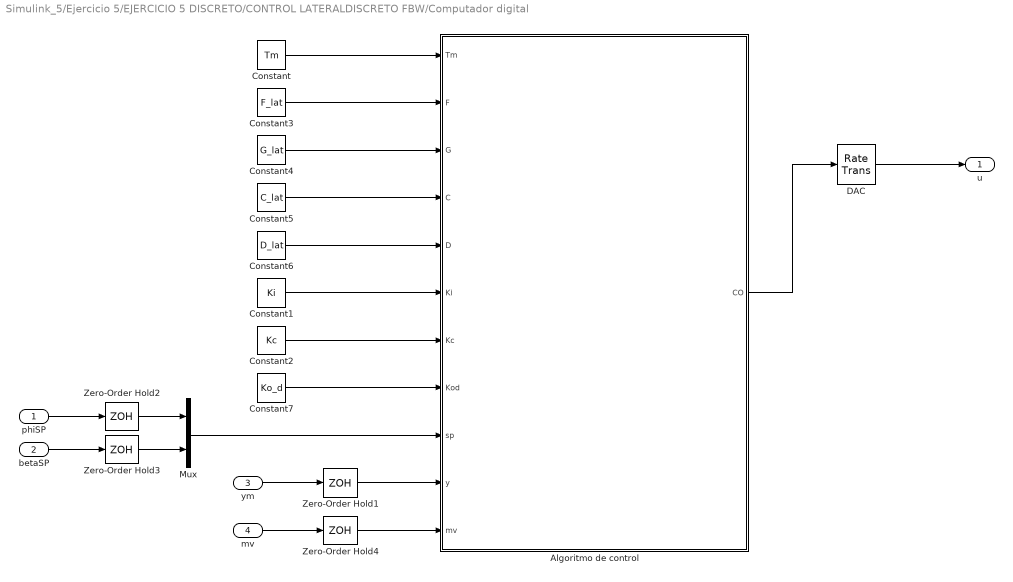
== system Simulink_5/Ejercicio 5/EJERCICIO 5 DISCRETO/CONTROL LATERALDISCRETO FBW/Computador digital ==
  phiSP : Inport
  betaSP : Inport  Port=2
  ym : Inport  Port=3
  mv : Inport  Port=4
  Algoritmo de control : MATLAB Function  TreatAsAtomicUnit=on
  Constant : Constant  Value=Tm
  Constant1 : Constant  Value=Ki
  Constant2 : Constant  Value=Kc
  Constant3 : Constant  Value=F_lat
  Constant4 : Constant  Value=G_lat
  Constant5 : Constant  Value=C_lat
  Constant6 : Constant  Value=D_lat
  Constant7 : Constant  Value=Ko_d
  DAC : RateTransition
  Mux : Mux  Inputs=2
  Zero-Order Hold{1..4} (4 alike) : ZeroOrderHold  SampleTime=Tm
  u : Outport
  wires:
  ym/1 -> Zero-Order Hold1/1
  mv/1 -> Zero-Order Hold4/1
  Constant7/1 -> Algoritmo de control/8(Kod)
  Constant6/1 -> Algoritmo de control/5(D)
  Constant5/1 -> Algoritmo de control/4(C)
  Constant4/1 -> Algoritmo de control/3(G)
  Constant3/1 -> Algoritmo de control/2(F)
  Constant2/1 -> Algoritmo de control/7(Kc)
  Constant/1 -> Algoritmo de control/1(Tm)
  Algoritmo de control/1(CO) -> DAC/1
  DAC/1 -> u/1
  phiSP/1 -> Zero-Order Hold2/1
  betaSP/1 -> Zero-Order Hold3/1
  Zero-Order Hold1/1 -> Algoritmo de control/10(y)
  Zero-Order Hold4/1 -> Algoritmo de control/11(mv)
  Zero-Order Hold2/1 -> Mux/1
  Zero-Order Hold3/1 -> Mux/2
  Mux/1 -> Algoritmo de control/9(sp)
  Constant1/1 -> Algoritmo de control/6(Ki)

== system Simulink_5/Ejercicio 5/EJERCICIO 5 DISCRETO/CONTROL LATERALDISCRETO FBW/Dinamica Lateral1 ==
  u : Inport
  Integrator5 : Integrator
  Km1 : Gain  Gain=D  Multiplication=Matrix(K*u)
  Km10 : Gain  Gain=A  Multiplication=Matrix(K*u)
  Km2 : Gain  Gain=C  Multiplication=Matrix(K*u)
  Km8 : Gain  Gain=B  Multiplication=Matrix(K*u)
  Sum1 : Sum  Inputs=++|
  Sum12 : Sum  Inputs=|++
  y : Outport
  wires:
  Km8/1 -> Sum12/1
  Sum12/1 -> Integrator5/1
  Integrator5/1 -> Km10/1, Km2/1  "x"
  Km10/1 -> Sum12/2
  Km2/1 -> Sum1/2
  Km1/1 -> Sum1/1
  Sum1/1 -> y/1
  u/1 -> Km8/1, Km1/1

== system Simulink_5/Ejercicio 5/EJERCICIO 5 DISCRETO/CONTROL LATERALDISCRETO FBW/SENSORES ==
  y : Inport
  Add2 : Sum
  Add3 : Sum
  Demux : Demux  Outputs=2
  Mux2 : Mux  Inputs=2
  Ruido de medida1 : RandomNumber  Variance=1e-6  Seed=123456  SampleTime=dt
  Ruido de medida2 : RandomNumber  Variance=1e-6  Seed=123456  SampleTime=dt
  ym : Outport
  wires:
  y/1 -> Demux/1
  Ruido de medida1/1 -> Add2/1
  Add2/1 -> Mux2/1
  Demux/1 -> Add2/2
  Mux2/1 -> ym/1
  Demux/2 -> Add3/1
  Add3/1 -> Mux2/2
  Ruido de medida2/1 -> Add3/2

== system Simulink_5/Ejercicio 5/EJERCICIO 5 CONTINUO/Control lateral con observador de estados %bien/Actuadores/Aleron ==
  u_a : Inport
  Transfer Fcn : TransferFcn  Numerator=[1/tau_a]  Denominator=[1 1/tau_a]
  delta_a : Outport
  wires:
  u_a/1 -> Transfer Fcn/1
  Transfer Fcn/1 -> delta_a/1

== system Simulink_5/Ejercicio 5/EJERCICIO 5 CONTINUO/Control lateral con observador de estados %bien/Actuadores/TIMÓN ==
  u_r : Inport
  Transfer Fcn : TransferFcn  Numerator=[1/tau_r]  Denominator=[1 1/tau_r]
  delta_r : Outport
  wires:
  u_r/1 -> Transfer Fcn/1
  Transfer Fcn/1 -> delta_r/1

== system Simulink_5/Ejercicio 5/EJERCICIO 5 CONTINUO/Control lateral con observador de estados sin perturbacion %bien/Actuadores/Aleron ==
  u_a : Inport
  Transfer Fcn : TransferFcn  Numerator=[1/tau_a]  Denominator=[1 1/tau_a]
  delta_a : Outport
  wires:
  u_a/1 -> Transfer Fcn/1
  Transfer Fcn/1 -> delta_a/1

== system Simulink_5/Ejercicio 5/EJERCICIO 5 CONTINUO/Control lateral con observador de estados sin perturbacion %bien/Actuadores/TIMÓN ==
  u_r : Inport
  Transfer Fcn : TransferFcn  Numerator=[1/tau_r]  Denominator=[1 1/tau_r]
  delta_r : Outport
  wires:
  u_r/1 -> Transfer Fcn/1
  Transfer Fcn/1 -> delta_r/1

== system Simulink_5/Ejercicio 5/EJERCICIO 5 CONTINUO/Control laterall con accion integral %bien/Actuadores/Aleron ==
  u_a : Inport
  Transfer Fcn : TransferFcn  Numerator=[1/tau_a]  Denominator=[1 1/tau_a]
  delta_a : Outport
  wires:
  u_a/1 -> Transfer Fcn/1
  Transfer Fcn/1 -> delta_a/1

== system Simulink_5/Ejercicio 5/EJERCICIO 5 CONTINUO/Control laterall con accion integral %bien/Actuadores/TIMÓN ==
  u_r : Inport
  Transfer Fcn : TransferFcn  Numerator=[1/tau_r]  Denominator=[1 1/tau_r]
  delta_r : Outport
  wires:
  u_r/1 -> Transfer Fcn/1
  Transfer Fcn/1 -> delta_r/1

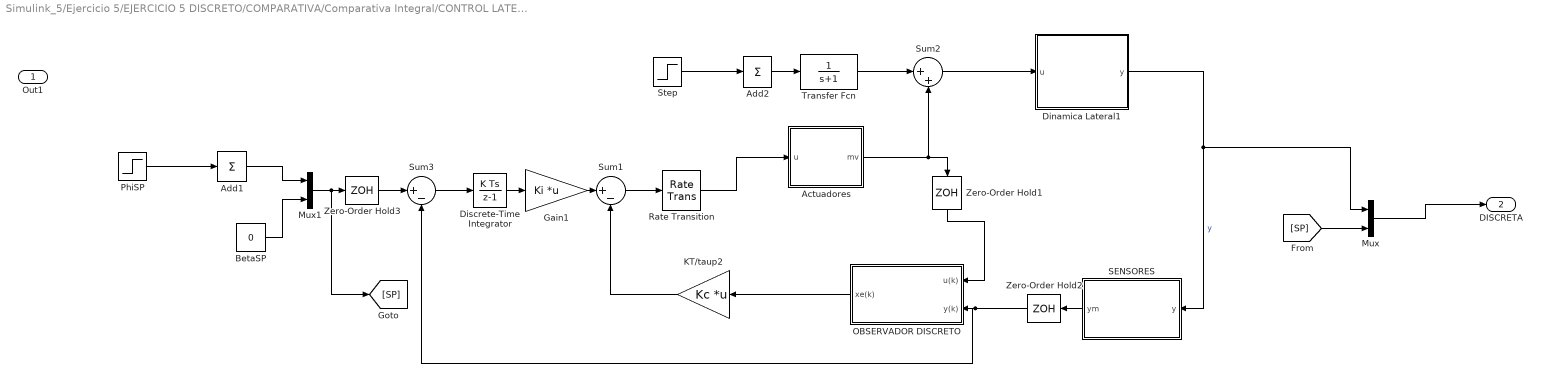
== system Simulink_5/Ejercicio 5/EJERCICIO 5 DISCRETO/COMPARATIVA/Comparativa Integral/CONTROL LATERAL DISCRETO ACCION INTEGRAL %bien ==
  Actuadores : Subsystem
  Add1 : Sum  Inputs=+
  Add2 : Sum  Inputs=+
  BetaSP : Constant  Value=0
  Dinamica Lateral1 : Subsystem  mask(Dinámica longitudinal F-16){A=sys_lat.a, B=sys_lat.b, C=sys_lat.c, D=sys_lat.d, X0=[0 0 0 0]}
      mask prompts: A "Matriz de estados (A)"; B "Matriz de entrada (B)"; C "Matriz de salida (C)"; D "Matriz de transmisión directa (D)"; X0 "Condiciones iniciales (nominales)"
      mask help: Modelo lineal de la dinámica longitudinal del F-16
  Discrete-Time Integrator : DiscreteIntegrator  InitialConditionSetting=State (most efficient)  SampleTime=-1  ICPrevOutput=DiscIntNeverNeededParam  ICPrevScaledInput=DiscIntNeverNeededParam
  Gain1 : Gain  Gain=Ki  Multiplication=Matrix(K*u)
  KT/taup2 : Gain  Gain=Kc  Multiplication=Matrix(K*u)
  Mux : Mux  Inputs=2
  Mux1 : Mux  Inputs=2
  OBSERVADOR DISCRETO : Subsystem  mask(Dinámica longitudinal F-16){F=F_lat, G=G_lat, C=C_lat, D=D_lat, Ko=Ko_d}
      mask prompts: F "Matriz de estados (A)"; G "Matriz de entrada (B)"; C "Matriz de salida (C)"; D "Matriz de transmisión directa (D)"; Ko "Ganancia del observador"
      mask help: Modelo lineal de la dinámica longitudinal del F-16
  PhiSP : Step  Time=[5 25]  Before=[0 0]  After=[10 -10]  SampleTime=0
  Rate Transition : RateTransition
  SENSORES : Subsystem
  Step : Step  Time=[40 41]  After=[1 -1]  SampleTime=0
  Sum1 : Sum  Inputs=|+-
  Sum2 : Sum  Inputs=|++
  Sum3 : Sum  Inputs=|+-
  Transfer Fcn : TransferFcn  Denominator=[1 1]
  Zero-Order Hold1 : ZeroOrderHold  SampleTime=-1
  Zero-Order Hold2 : ZeroOrderHold  SampleTime=-1
  Zero-Order Hold3 : ZeroOrderHold  SampleTime=-1
  Out1 : Outport
  DISCRETA : Outport  Port=2
  wires:
  Zero-Order Hold2/1 -> Sum3/2, OBSERVADOR DISCRETO/2(y(k))
  Rate Transition/1 -> Actuadores/1(u)
  Mux1/1 -> Zero-Order Hold3/1, [SP]
  Dinamica Lateral1/1(y) -> SENSORES/1(y), Mux/1  "y"
  [SP] -> Mux/2
  Add2/1 -> Transfer Fcn/1
  Gain1/1 -> Sum1/1
  Discrete-Time Integrator/1 -> Gain1/1
  SENSORES/1(ym) -> Zero-Order Hold2/1
  Transfer Fcn/1 -> Sum2/1
  Step/1 -> Add2/1
  KT/taup2/1 -> Sum1/2
  BetaSP/1 -> Mux1/2
  Sum1/1 -> Rate Transition/1
  OBSERVADOR DISCRETO/1(xe(k)) -> KT/taup2/1
  Add1/1 -> Mux1/1
  Actuadores/1(mv) -> Zero-Order Hold1/1, Sum2/2
  PhiSP/1 -> Add1/1
  Mux/1 -> DISCRETA/1
  Sum2/1 -> Dinamica Lateral1/1(u)
  Zero-Order Hold1/1 -> OBSERVADOR DISCRETO/1(u(k))
  Sum3/1 -> Discrete-Time Integrator/1
  Zero-Order Hold3/1 -> Sum3/1

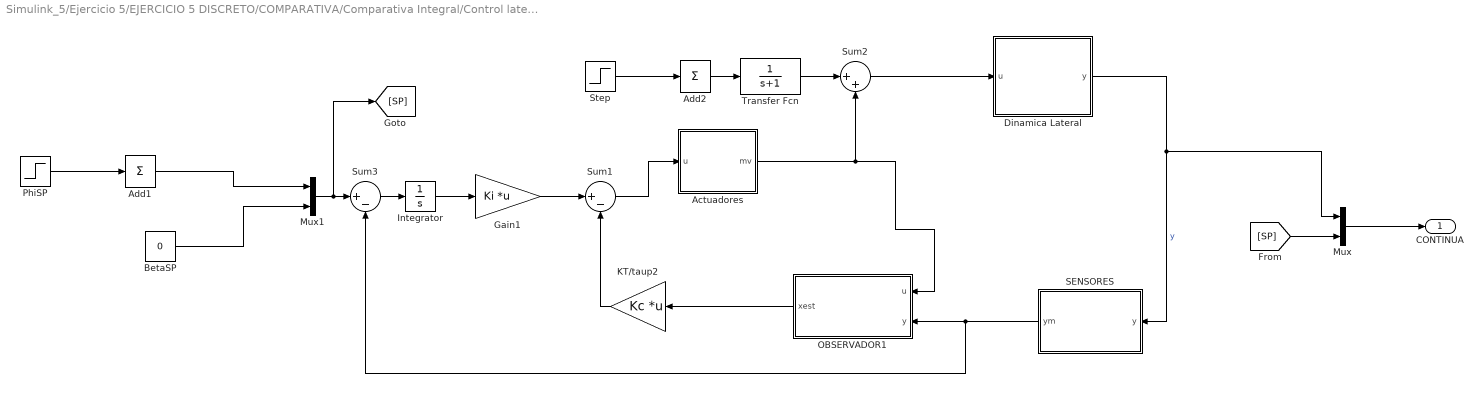
== system Simulink_5/Ejercicio 5/EJERCICIO 5 DISCRETO/COMPARATIVA/Comparativa Integral/Control laterall con accion integral %bien ==
  Actuadores : Subsystem
  Add1 : Sum  Inputs=+
  Add2 : Sum  Inputs=+
  BetaSP : Constant  Value=0
  Dinamica Lateral : Subsystem  mask(Dinámica longitudinal F-16){A=sys_lat.a, B=sys_lat.b, C=sys_lat.c, D=sys_lat.d, X0=[0 0 0 0]}
      mask prompts: A "Matriz de estados (A)"; B "Matriz de entrada (B)"; C "Matriz de salida (C)"; D "Matriz de transmisión directa (D)"; X0 "Condiciones iniciales (nominales)"
      mask help: Modelo lineal de la dinámica longitudinal del F-16
  Gain1 : Gain  Gain=Ki  Multiplication=Matrix(K*u)
  Integrator : Integrator
  KT/taup2 : Gain  Gain=Kc  Multiplication=Matrix(K*u)
  Mux : Mux  Inputs=2
  Mux1 : Mux  Inputs=2
  OBSERVADOR1 : Subsystem  mask(Dinámica longitudinal F-16){A=sys_lat.a, B=sys_lat.b, C=sys_lat.c, D=sys_lat.d, X0=[0 0 0 0], Ko=Ko}
      mask prompts: A "Matriz de estados (A)"; B "Matriz de entrada (B)"; C "Matriz de salida (C)"; D "Matriz de transmisión directa (D)"; X0 "Condiciones iniciales (nominales)"; Ko "Ganancia del observador"
      mask help: Modelo lineal de la dinámica longitudinal del F-16
  PhiSP : Step  Time=[5 25]  Before=[0 0]  After=[10 -10]  SampleTime=0
  SENSORES : Subsystem
  Step : Step  Time=[40 41]  After=[1 -1]  SampleTime=0
  Sum1 : Sum  Inputs=|+-
  Sum2 : Sum  Inputs=|++
  Sum3 : Sum  Inputs=|+-
  Transfer Fcn : TransferFcn  Denominator=[1 1]
  CONTINUA : Outport
  wires:
  Actuadores/1(mv) -> OBSERVADOR1/1(u), Sum2/2
  Dinamica Lateral/1(y) -> Mux/1, SENSORES/1(y)  "y"
  BetaSP/1 -> Mux1/2
  Add1/1 -> Mux1/1
  Sum2/1 -> Dinamica Lateral/1(u)
  KT/taup2/1 -> Sum1/2
  Gain1/1 -> Sum1/1
  Add2/1 -> Transfer Fcn/1
  Step/1 -> Add2/1
  PhiSP/1 -> Add1/1
  SENSORES/1(ym) -> OBSERVADOR1/2(y), Sum3/2
  Mux/1 -> CONTINUA/1
  Sum1/1 -> Actuadores/1(u)
  [SP] -> Mux/2
  OBSERVADOR1/1(xest) -> KT/taup2/1
  Transfer Fcn/1 -> Sum2/1
  Mux1/1 -> [SP], Sum3/1
  Integrator/1 -> Gain1/1
  Sum3/1 -> Integrator/1

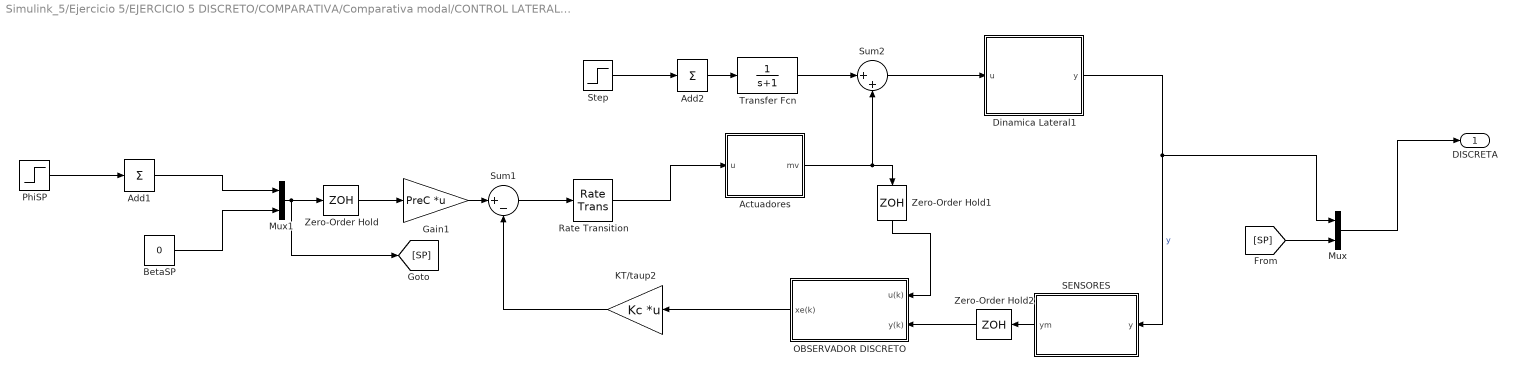
== system Simulink_5/Ejercicio 5/EJERCICIO 5 DISCRETO/COMPARATIVA/Comparativa modal/CONTROL LATERAL DISCRETO %bien ==
  Actuadores : Subsystem
  Add1 : Sum  Inputs=+
  Add2 : Sum  Inputs=+
  BetaSP : Constant  Value=0
  Dinamica Lateral1 : Subsystem  mask(Dinámica longitudinal F-16){A=sys_lat.a, B=sys_lat.b, C=sys_lat.c, D=sys_lat.d, X0=[0 0 0 0]}
      mask prompts: A "Matriz de estados (A)"; B "Matriz de entrada (B)"; C "Matriz de salida (C)"; D "Matriz de transmisión directa (D)"; X0 "Condiciones iniciales (nominales)"
      mask help: Modelo lineal de la dinámica longitudinal del F-16
  Gain1 : Gain  Gain=PreC  Multiplication=Matrix(K*u)
  KT/taup2 : Gain  Gain=Kc  Multiplication=Matrix(K*u)
  Mux : Mux  Inputs=2
  Mux1 : Mux  Inputs=2
  OBSERVADOR DISCRETO : Subsystem  mask(Dinámica longitudinal F-16){F=F_lat, G=G_lat, C=C_lat, D=D_lat, Ko=Ko_d}
      mask prompts: F "Matriz de estados (A)"; G "Matriz de entrada (B)"; C "Matriz de salida (C)"; D "Matriz de transmisión directa (D)"; Ko "Ganancia del observador"
      mask help: Modelo lineal de la dinámica longitudinal del F-16
  PhiSP : Step  Time=[5 25]  Before=[0 0]  After=[10 -10]  SampleTime=0
  Rate Transition : RateTransition
  SENSORES : Subsystem
  Step : Step  Time=[40 41]  After=[1 -1]  SampleTime=0
  Sum1 : Sum  Inputs=|+-
  Sum2 : Sum  Inputs=|++
  Transfer Fcn : TransferFcn  Denominator=[1 1]
  Zero-Order Hold : ZeroOrderHold  SampleTime=-1
  Zero-Order Hold1 : ZeroOrderHold  SampleTime=-1
  Zero-Order Hold2 : ZeroOrderHold  SampleTime=-1
  DISCRETA : Outport
  wires:
  Actuadores/1(mv) -> Zero-Order Hold1/1, Sum2/2
  Mux1/1 -> Zero-Order Hold/1, [SP]
  [SP] -> Mux/2
  Add1/1 -> Mux1/1
  OBSERVADOR DISCRETO/1(xe(k)) -> KT/taup2/1
  SENSORES/1(ym) -> Zero-Order Hold2/1
  KT/taup2/1 -> Sum1/2
  PhiSP/1 -> Add1/1
  Gain1/1 -> Sum1/1
  Mux/1 -> DISCRETA/1
  BetaSP/1 -> Mux1/2
  Dinamica Lateral1/1(y) -> SENSORES/1(y), Mux/1  "y"
  Zero-Order Hold/1 -> Gain1/1
  Rate Transition/1 -> Actuadores/1(u)
  Sum1/1 -> Rate Transition/1
  Zero-Order Hold1/1 -> OBSERVADOR DISCRETO/1(u(k))
  Zero-Order Hold2/1 -> OBSERVADOR DISCRETO/2(y(k))
  Add2/1 -> Transfer Fcn/1
  Step/1 -> Add2/1
  Transfer Fcn/1 -> Sum2/1
  Sum2/1 -> Dinamica Lateral1/1(u)

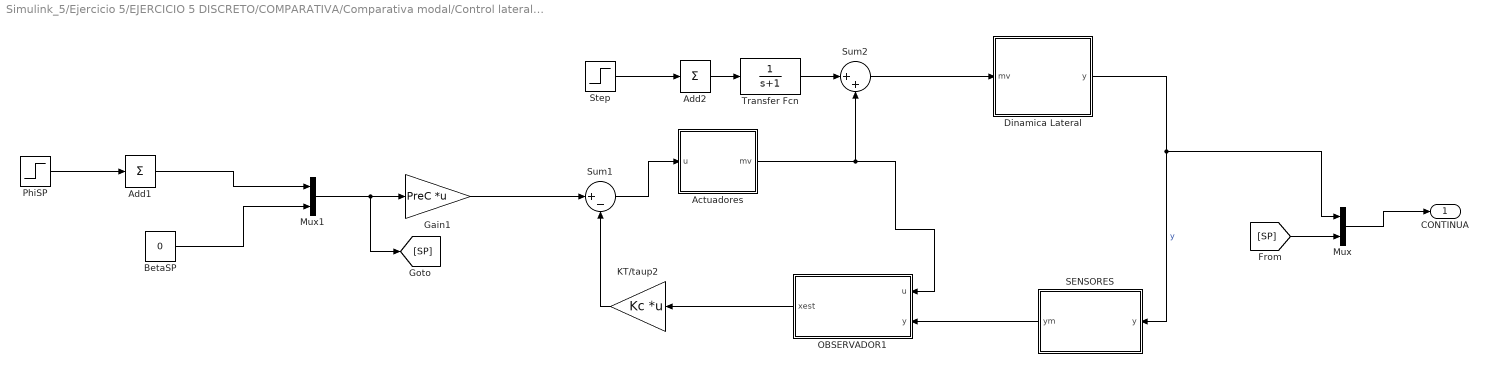
== system Simulink_5/Ejercicio 5/EJERCICIO 5 DISCRETO/COMPARATIVA/Comparativa modal/Control lateral con observador de estados %bien ==
  Actuadores : Subsystem
  Add1 : Sum  Inputs=+
  Add2 : Sum  Inputs=+
  BetaSP : Constant  Value=0
  Dinamica Lateral : Subsystem  mask(Dinámica longitudinal F-16){A=sys_lat.a, B=sys_lat.b, C=sys_lat.c, D=sys_lat.d, X0=[0 0 0 0]}
      mask prompts: A "Matriz de estados (A)"; B "Matriz de entrada (B)"; C "Matriz de salida (C)"; D "Matriz de transmisión directa (D)"; X0 "Condiciones iniciales (nominales)"
      mask help: Modelo lineal de la dinámica longitudinal del F-16
  Gain1 : Gain  Gain=PreC  Multiplication=Matrix(K*u)
  KT/taup2 : Gain  Gain=Kc  Multiplication=Matrix(K*u)
  Mux : Mux  Inputs=2
  Mux1 : Mux  Inputs=2
  OBSERVADOR1 : Subsystem  mask(Dinámica longitudinal F-16){A=sys_lat.a, B=sys_lat.b, C=sys_lat.c, D=sys_lat.d, X0=[0 0 0 0], Ko=Ko}
      mask prompts: A "Matriz de estados (A)"; B "Matriz de entrada (B)"; C "Matriz de salida (C)"; D "Matriz de transmisión directa (D)"; X0 "Condiciones iniciales (nominales)"; Ko "Ganancia del observador"
      mask help: Modelo lineal de la dinámica longitudinal del F-16
  PhiSP : Step  Time=[5 25]  Before=[0 0]  After=[10 -10]  SampleTime=0
  SENSORES : Subsystem
  Step : Step  Time=[40 41]  After=[1 -1]  SampleTime=0
  Sum1 : Sum  Inputs=|+-
  Sum2 : Sum  Inputs=|++
  Transfer Fcn : TransferFcn  Denominator=[1 1]
  CONTINUA : Outport
  wires:
  Mux1/1 -> [SP], Gain1/1
  Gain1/1 -> Sum1/1
  Mux/1 -> CONTINUA/1
  [SP] -> Mux/2
  KT/taup2/1 -> Sum1/2
  SENSORES/1(ym) -> OBSERVADOR1/2(y)
  OBSERVADOR1/1(xest) -> KT/taup2/1
  Dinamica Lateral/1(y) -> Mux/1, SENSORES/1(y)  "y"
  PhiSP/1 -> Add1/1
  Add1/1 -> Mux1/1
  Actuadores/1(mv) -> OBSERVADOR1/1(u), Sum2/2
  Sum1/1 -> Actuadores/1(u)
  BetaSP/1 -> Mux1/2
  Step/1 -> Add2/1
  Transfer Fcn/1 -> Sum2/1
  Add2/1 -> Transfer Fcn/1
  Sum2/1 -> Dinamica Lateral/1(mv)

== system Simulink_5/Ejercicio 5/EJERCICIO 5 DISCRETO/CONTROL LATERAL DISCRETO/Actuadores/Aleron ==
  u_a : Inport
  Transfer Fcn : TransferFcn  Numerator=[1/tau_a]  Denominator=[1 1/tau_a]
  delta_a : Outport
  wires:
  u_a/1 -> Transfer Fcn/1
  Transfer Fcn/1 -> delta_a/1

== system Simulink_5/Ejercicio 5/EJERCICIO 5 DISCRETO/CONTROL LATERAL DISCRETO/Actuadores/TIMÓN ==
  u_r : Inport
  Transfer Fcn : TransferFcn  Numerator=[1/tau_r]  Denominator=[1 1/tau_r]
  delta_r : Outport
  wires:
  u_r/1 -> Transfer Fcn/1
  Transfer Fcn/1 -> delta_r/1

== system Simulink_5/Ejercicio 5/EJERCICIO 5 DISCRETO/CONTROL LATERAL DISCRETO ACCION INTEGRAL/Actuadores/Aleron ==
  u_a : Inport
  Transfer Fcn : TransferFcn  Numerator=[1/tau_a]  Denominator=[1 1/tau_a]
  delta_a : Outport
  wires:
  u_a/1 -> Transfer Fcn/1
  Transfer Fcn/1 -> delta_a/1

== system Simulink_5/Ejercicio 5/EJERCICIO 5 DISCRETO/CONTROL LATERAL DISCRETO ACCION INTEGRAL/Actuadores/TIMÓN ==
  u_r : Inport
  Transfer Fcn : TransferFcn  Numerator=[1/tau_r]  Denominator=[1 1/tau_r]
  delta_r : Outport
  wires:
  u_r/1 -> Transfer Fcn/1
  Transfer Fcn/1 -> delta_r/1

== system Simulink_5/Ejercicio 5/EJERCICIO 5 DISCRETO/CONTROL LATERALDISCRETO FBW/Actuadores/Aleron ==
  u_a : Inport
  Transfer Fcn : TransferFcn  Numerator=[1/tau_a]  Denominator=[1 1/tau_a]
  delta_a : Outport
  wires:
  u_a/1 -> Transfer Fcn/1
  Transfer Fcn/1 -> delta_a/1

== system Simulink_5/Ejercicio 5/EJERCICIO 5 DISCRETO/CONTROL LATERALDISCRETO FBW/Actuadores/TIMÓN ==
  u_r : Inport
  Transfer Fcn : TransferFcn  Numerator=[1/tau_r]  Denominator=[1 1/tau_r]
  delta_r : Outport
  wires:
  u_r/1 -> Transfer Fcn/1
  Transfer Fcn/1 -> delta_r/1

== system Simulink_5/Ejercicio 5/EJERCICIO 5 DISCRETO/COMPARATIVA/Comparativa Integral/CONTROL LATERAL DISCRETO ACCION INTEGRAL %bien/Actuadores ==
  u : Inport
  Aleron : Subsystem
  Demux : Demux  Outputs=2
  Mux2 : Mux  Inputs=2
  Scope : Scope
  TIMÓN : Subsystem
  mv : Outport
  wires:
  u/1 -> Demux/1
  Mux2/1 -> mv/1, Scope/1
  Demux/1 -> Aleron/1(u_a)
  Demux/2 -> TIMÓN/1(u_r)
  Aleron/1(delta_a) -> Mux2/1
  TIMÓN/1(delta_r) -> Mux2/2

== system Simulink_5/Ejercicio 5/EJERCICIO 5 DISCRETO/COMPARATIVA/Comparativa Integral/CONTROL LATERAL DISCRETO ACCION INTEGRAL %bien/Dinamica Lateral1 ==
  u : Inport
  Integrator5 : Integrator
  Km1 : Gain  Gain=D  Multiplication=Matrix(K*u)
  Km10 : Gain  Gain=A  Multiplication=Matrix(K*u)
  Km2 : Gain  Gain=C  Multiplication=Matrix(K*u)
  Km8 : Gain  Gain=B  Multiplication=Matrix(K*u)
  Sum1 : Sum  Inputs=++|
  Sum12 : Sum  Inputs=|++
  y : Outport
  wires:
  Km8/1 -> Sum12/1
  Sum12/1 -> Integrator5/1
  Integrator5/1 -> Km10/1, Km2/1  "x"
  Km10/1 -> Sum12/2
  Km2/1 -> Sum1/2
  Km1/1 -> Sum1/1
  Sum1/1 -> y/1
  u/1 -> Km8/1, Km1/1

== system Simulink_5/Ejercicio 5/EJERCICIO 5 DISCRETO/COMPARATIVA/Comparativa Integral/CONTROL LATERAL DISCRETO ACCION INTEGRAL %bien/OBSERVADOR DISCRETO ==
  u(k) : Inport
  y(k) : Inport  Port=2
  Km1 : Gain  Gain=D  Multiplication=Matrix(K*u)
  Km10 : Gain  Gain=F  Multiplication=Matrix(K*u)
  Km2 : Gain  Gain=C  Multiplication=Matrix(K*u)
  Km3 : Gain  Gain=Ko  Multiplication=Matrix(K*u)
  Km8 : Gain  Gain=G  Multiplication=Matrix(K*u)
  Sum1 : Sum  Inputs=++|
  Sum12 : Sum  Inputs=+++
  Sum2 : Sum  Inputs=+-|
  Unit Delay : UnitDelay  SampleTime=Tm  HasFrameUpgradeWarning=on
  xe(k) : Outport
  wires:
  Km8/1 -> Sum12/1
  Sum12/1 -> Unit Delay/1  "xe(k+1)"
  Unit Delay/1 -> Km2/1, Km10/1, xe(k)/1  "xe(k)"
  Km10/1 -> Sum12/3
  Km2/1 -> Sum1/2
  Km1/1 -> Sum1/1
  Sum1/1 -> Sum2/2  "ye(k)"
  u(k)/1 -> Km8/1, Km1/1
  y(k)/1 -> Sum2/1
  Sum2/1 -> Km3/1
  Km3/1 -> Sum12/2

== system Simulink_5/Ejercicio 5/EJERCICIO 5 DISCRETO/COMPARATIVA/Comparativa Integral/CONTROL LATERAL DISCRETO ACCION INTEGRAL %bien/SENSORES ==
  y : Inport
  Add2 : Sum
  Add3 : Sum
  Demux : Demux  Outputs=2
  Mux2 : Mux  Inputs=2
  Ruido de medida1 : RandomNumber  Variance=1e-6  Seed=123456  SampleTime=dt
  Ruido de medida2 : RandomNumber  Variance=1e-6  Seed=123456  SampleTime=dt
  ym : Outport
  wires:
  y/1 -> Demux/1
  Ruido de medida1/1 -> Add2/1
  Add2/1 -> Mux2/1
  Demux/1 -> Add2/2
  Mux2/1 -> ym/1
  Demux/2 -> Add3/1
  Add3/1 -> Mux2/2
  Ruido de medida2/1 -> Add3/2

== system Simulink_5/Ejercicio 5/EJERCICIO 5 DISCRETO/COMPARATIVA/Comparativa Integral/Control laterall con accion integral %bien/Actuadores ==
  u : Inport
  Aleron : Subsystem
  Demux : Demux  Outputs=2
  Mux2 : Mux  Inputs=2
  Scope : Scope
  TIMÓN : Subsystem
  mv : Outport
  wires:
  u/1 -> Demux/1
  Mux2/1 -> mv/1, Scope/1
  Demux/1 -> Aleron/1(u_a)
  Demux/2 -> TIMÓN/1(u_r)
  Aleron/1(delta_a) -> Mux2/1
  TIMÓN/1(delta_r) -> Mux2/2

== system Simulink_5/Ejercicio 5/EJERCICIO 5 DISCRETO/COMPARATIVA/Comparativa Integral/Control laterall con accion integral %bien/Dinamica Lateral ==
  u : Inport
  Integrator5 : Integrator
  Km1 : Gain  Gain=D  Multiplication=Matrix(K*u)
  Km10 : Gain  Gain=A  Multiplication=Matrix(K*u)
  Km2 : Gain  Gain=C  Multiplication=Matrix(K*u)
  Km8 : Gain  Gain=B  Multiplication=Matrix(K*u)
  Sum1 : Sum  Inputs=++|
  Sum12 : Sum  Inputs=|++
  y : Outport
  wires:
  Km8/1 -> Sum12/1
  Sum12/1 -> Integrator5/1
  Integrator5/1 -> Km10/1, Km2/1  "x"
  Km10/1 -> Sum12/2
  Km2/1 -> Sum1/2
  Km1/1 -> Sum1/1
  Sum1/1 -> y/1
  u/1 -> Km8/1, Km1/1

== system Simulink_5/Ejercicio 5/EJERCICIO 5 DISCRETO/COMPARATIVA/Comparativa Integral/Control laterall con accion integral %bien/OBSERVADOR1 ==
  u : Inport
  y : Inport  Port=2
  Integrator5 : Integrator
  Km1 : Gain  Gain=D  Multiplication=Matrix(K*u)
  Km10 : Gain  Gain=A  Multiplication=Matrix(K*u)
  Km2 : Gain  Gain=C  Multiplication=Matrix(K*u)
  Km3 : Gain  Gain=Ko  Multiplication=Matrix(K*u)
  Km8 : Gain  Gain=B  Multiplication=Matrix(K*u)
  Sum1 : Sum  Inputs=++|
  Sum12 : Sum  Inputs=+++
  Sum2 : Sum  Inputs=+-|
  xest : Outport
  wires:
  Km8/1 -> Sum12/1
  Sum12/1 -> Integrator5/1
  Integrator5/1 -> Km2/1, Km10/1, xest/1  "xe"
  Km10/1 -> Sum12/3
  Km2/1 -> Sum1/2
  Km1/1 -> Sum1/1
  Sum1/1 -> Sum2/2  "ye"
  u/1 -> Km8/1, Km1/1
  y/1 -> Sum2/1
  Sum2/1 -> Km3/1
  Km3/1 -> Sum12/2

== system Simulink_5/Ejercicio 5/EJERCICIO 5 DISCRETO/COMPARATIVA/Comparativa Integral/Control laterall con accion integral %bien/SENSORES ==
  y : Inport
  Add2 : Sum
  Add3 : Sum
  Demux : Demux  Outputs=2
  Mux2 : Mux  Inputs=2
  Ruido de medida1 : RandomNumber  Variance=1e-6  Seed=123456  SampleTime=dt
  Ruido de medida2 : RandomNumber  Variance=1e-6  Seed=123456  SampleTime=dt
  ym : Outport
  wires:
  y/1 -> Demux/1
  Ruido de medida1/1 -> Add2/1
  Add2/1 -> Mux2/1
  Demux/1 -> Add2/2
  Mux2/1 -> ym/1
  Demux/2 -> Add3/1
  Add3/1 -> Mux2/2
  Ruido de medida2/1 -> Add3/2

== system Simulink_5/Ejercicio 5/EJERCICIO 5 DISCRETO/COMPARATIVA/Comparativa modal/CONTROL LATERAL DISCRETO %bien/Actuadores ==
  u : Inport
  Aleron : Subsystem
  Demux : Demux  Outputs=2
  Mux2 : Mux  Inputs=2
  Scope : Scope
  TIMÓN : Subsystem
  mv : Outport
  wires:
  u/1 -> Demux/1
  Mux2/1 -> mv/1, Scope/1
  Demux/1 -> Aleron/1(u_a)
  Demux/2 -> TIMÓN/1(u_r)
  Aleron/1(delta_a) -> Mux2/1
  TIMÓN/1(delta_r) -> Mux2/2

== system Simulink_5/Ejercicio 5/EJERCICIO 5 DISCRETO/COMPARATIVA/Comparativa modal/CONTROL LATERAL DISCRETO %bien/Dinamica Lateral1 ==
  u : Inport
  Integrator5 : Integrator
  Km1 : Gain  Gain=D  Multiplication=Matrix(K*u)
  Km10 : Gain  Gain=A  Multiplication=Matrix(K*u)
  Km2 : Gain  Gain=C  Multiplication=Matrix(K*u)
  Km8 : Gain  Gain=B  Multiplication=Matrix(K*u)
  Sum1 : Sum  Inputs=++|
  Sum12 : Sum  Inputs=|++
  y : Outport
  wires:
  Km8/1 -> Sum12/1
  Sum12/1 -> Integrator5/1
  Integrator5/1 -> Km10/1, Km2/1  "x"
  Km10/1 -> Sum12/2
  Km2/1 -> Sum1/2
  Km1/1 -> Sum1/1
  Sum1/1 -> y/1
  u/1 -> Km8/1, Km1/1

== system Simulink_5/Ejercicio 5/EJERCICIO 5 DISCRETO/COMPARATIVA/Comparativa modal/CONTROL LATERAL DISCRETO %bien/OBSERVADOR DISCRETO ==
  u(k) : Inport
  y(k) : Inport  Port=2
  Km1 : Gain  Gain=D  Multiplication=Matrix(K*u)
  Km10 : Gain  Gain=F  Multiplication=Matrix(K*u)
  Km2 : Gain  Gain=C  Multiplication=Matrix(K*u)
  Km3 : Gain  Gain=Ko  Multiplication=Matrix(K*u)
  Km8 : Gain  Gain=G  Multiplication=Matrix(K*u)
  Sum1 : Sum  Inputs=++|
  Sum12 : Sum  Inputs=+++
  Sum2 : Sum  Inputs=+-|
  Unit Delay : UnitDelay  SampleTime=Tm  HasFrameUpgradeWarning=on
  xe(k) : Outport
  wires:
  Km8/1 -> Sum12/1
  Sum12/1 -> Unit Delay/1  "xe(k+1)"
  Unit Delay/1 -> Km2/1, Km10/1, xe(k)/1  "xe(k)"
  Km10/1 -> Sum12/3
  Km2/1 -> Sum1/2
  Km1/1 -> Sum1/1
  Sum1/1 -> Sum2/2  "ye(k)"
  u(k)/1 -> Km8/1, Km1/1
  y(k)/1 -> Sum2/1
  Sum2/1 -> Km3/1
  Km3/1 -> Sum12/2

== system Simulink_5/Ejercicio 5/EJERCICIO 5 DISCRETO/COMPARATIVA/Comparativa modal/CONTROL LATERAL DISCRETO %bien/SENSORES ==
  y : Inport
  Add2 : Sum
  Add3 : Sum
  Demux : Demux  Outputs=2
  Mux2 : Mux  Inputs=2
  Ruido de medida1 : RandomNumber  Variance=1e-6  Seed=123456  SampleTime=dt
  Ruido de medida2 : RandomNumber  Variance=1e-6  Seed=123456  SampleTime=dt
  ym : Outport
  wires:
  y/1 -> Demux/1
  Ruido de medida1/1 -> Add2/1
  Add2/1 -> Mux2/1
  Demux/1 -> Add2/2
  Mux2/1 -> ym/1
  Demux/2 -> Add3/1
  Add3/1 -> Mux2/2
  Ruido de medida2/1 -> Add3/2
